simulink model "boostConverter"  (R2021a)
settings: Solver=VariableStepAuto  StartTime=0.0  StopTime=2  RelTol=1e-3
model workspace (MAT data in the model file):
  C = Simulink.Parameter
  C.Value = 0.01
  C.DataType = 'auto'
  C.Dimensions = [1 1]
  L = Simulink.Parameter
  L.Value = 1e-05
  L.DataType = 'auto'
  L.Dimensions = [1 1]
  R = Simulink.Parameter
  R.Value = 10
  R.DataType = 'auto'
  R.Dimensions = [1 1]
libraries: spsSeriesRLCBranchLib x6, spsCurrentMeasurementLib x5, spsMosfetLib x3, spsVoltageMeasurementLib x3, spsControlledVoltageSourceLib x2, spsMeanLib x2, spsDiodeLib x1, simulink x1, spspowerguiLib x1
settings Model: Creator=User  LastModifiedBy=User

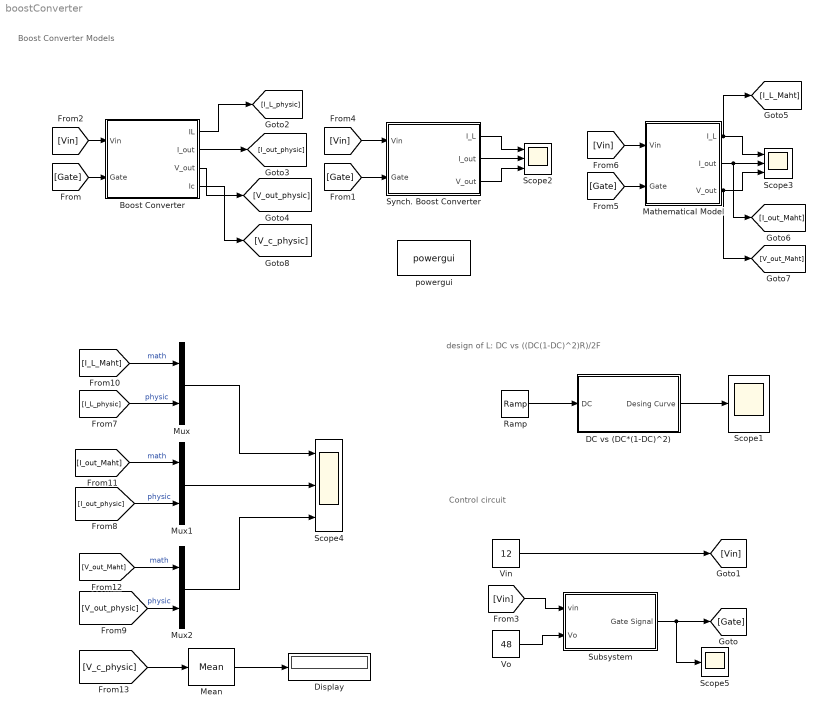
== system boostConverter ==
  note: Control circuit
  note: Boost Converter Models
  note: design of L: DC vs ((DC(1-DC)^2)R)/2F
  " DC vs (DC*(1-DC)^2) " : Subsystem  mask{F=50000, R=R, L=L}
  Boost Converter : Subsystem
  Display : Display
  Mathematical Model : Subsystem
  Mean : spsMeanLib/Mean  Freq=60  Vinit=0  Ts=0
  Mux : Mux  Inputs=2
  Mux1 : Mux  Inputs=2
  Mux2 : Mux  Inputs=2
  Ramp : simulink/Sources/Ramp  slope=1  start=0  InitialOutput=0
  Scope1 : Scope
  Scope2 : Scope  NumInputPorts=3
  Scope3 : Scope  NumInputPorts=3
  Scope4 : Scope  NumInputPorts=3
  Scope5 : Scope
  Subsystem : Subsystem
  Synch. Boost Converter : Subsystem
  Vin : Constant  Value=12
  Vo : Constant  Value=48
  powergui : spspowerguiLib/powergui  Priority=1  SimulationMode=Continuous  SampleTime=50e-6  frequency=60  Iterations=50  frequencyindice=0  Pbase=100e6  ErrMax=1e-4  UnitsV=kV  UnitsW=MW  buscounter=0  FunctionMessages=off  echomessages=off  EnableUseOfTLC=off  CurrentSourceSwitches=off  DisableSnubberDevices=on  DisableRonSwitches=off  DisableVfSwitches=off  DisplayEquations=off  AutomaticDiscreteSolvers=off  SolverType=Tustin/Backward Euler (TBE)  Interpol=off  ExternalGateDelay=off  methode=off  Ts=100  x0status=blocks  SPID=on  SwTol=0  HookPort=off  NonlinearTolerance=1e-4  nMaxIteration=100  ContinueOnMaxIteration=off  RestoreLinks=warning  ResistiveCurrentMeasurement=off  Frange=[0:2:500]  Ylog=off  Xlog=on  ShowGrid=off  save=off  variable=ZData  structure=0  ZoomFFT=off  StartTime=0.0  cycles=1  DisplayStyle=1  fundamental=60  FreqAxis=off  MaxFrequency=1000  frequencyindicesteady=1  RmsSteady=1  display=off
  wires:
  Vo/1 -> Subsystem/2(Vo)
  [Gate] -> Boost Converter/2(Gate)
  Ramp/1 -> " DC vs (DC*(1-DC)^2) "/1(DC)
  " DC vs (DC*(1-DC)^2) "/1(Desing Curve) -> Scope1/1
  Boost Converter/1(IL) -> [I_L_physic]
  [Gate] -> Synch. Boost Converter/2(Gate)
  Synch. Boost Converter/2(I_out) -> Scope2/2
  Synch. Boost Converter/1(I_L) -> Scope2/1
  Synch. Boost Converter/3(V_out) -> Scope2/3
  Vin/1 -> [Vin]
  [Vin] -> Boost Converter/1(Vin)
  [Vin] -> Subsystem/1(vin)
  [Vin] -> Synch. Boost Converter/1(Vin)
  [Gate] -> Mathematical Model/2(Gate)
  [Vin] -> Mathematical Model/1(Vin)
  Boost Converter/2(I_out) -> [I_out_physic]
  Boost Converter/3(V_out) -> [V_out_physic]
  Mathematical Model/1(I_L) -> [I_L_Maht], Scope3/1
  Mathematical Model/2(I_out) -> [I_out_Maht], Scope3/2
  Mathematical Model/3(V_out) -> [V_out_Maht], Scope3/3
  [I_L_Maht] -> Mux/1  "math"
  [I_L_physic] -> Mux/2  "physic"
  [I_out_Maht] -> Mux1/1  "math"
  [I_out_physic] -> Mux1/2  "physic"
  [V_out_Maht] -> Mux2/1  "math"
  [V_out_physic] -> Mux2/2  "physic"
  Mux/1 -> Scope4/1
  Mux1/1 -> Scope4/2
  Mux2/1 -> Scope4/3
  Subsystem/1(Gate Signal) -> Scope5/1, [Gate]
  Boost Converter/4(Ic) -> [V_c_physic]
  [V_c_physic] -> Mean/1
  Mean/1 -> Display/1

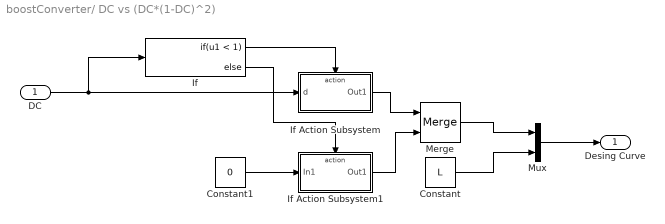
== system boostConverter/ DC vs (DC*(1-DC)^2)  ==
  DC : Inport
  Constant : Constant  Value=L
  Constant1 : Constant  Value=0
  If : If  IfExpression=u1 < 1
  If Action Subsystem : Subsystem  TreatAsAtomicUnit=on
  If Action Subsystem1 : Subsystem  TreatAsAtomicUnit=on
  Merge : Merge
  Mux : Mux  Inputs=2
  Desing Curve : Outport
  wires:
  Constant1/1 -> If Action Subsystem1/1(In1)
  If Action Subsystem/1(Out1) -> Merge/1
  If Action Subsystem1/1(Out1) -> Merge/2
  If/1 -> If Action Subsystem/Action
  DC/1 -> If/1, If Action Subsystem/1(d)
  If/2 -> If Action Subsystem1/Action
  Merge/1 -> Mux/1
  Constant/1 -> Mux/2
  Mux/1 -> Desing Curve/1

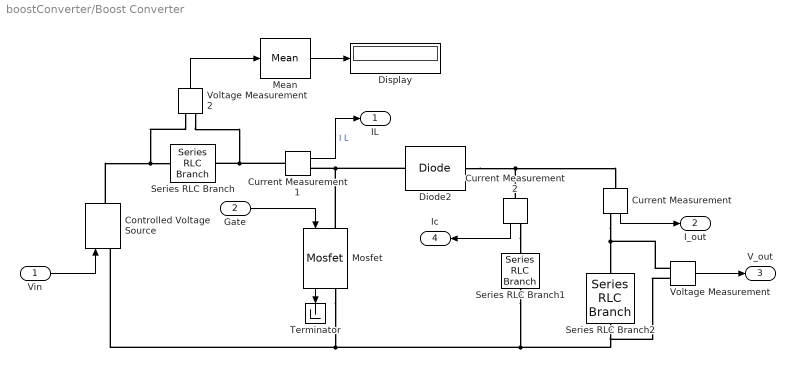
== system boostConverter/Boost Converter ==
  Vin : Inport
  Gate : Inport  Port=2
  Controlled Voltage Source : spsControlledVoltageSourceLib/Controlled Voltage Source  Initialize=on  Source_Type=AC  Amplitude=0  Phase=0  Frequency=0  Measurements=None
  Current Measurement : spsCurrentMeasurementLib/Current Measurement  PhasorSimulation=off  OutputType=Complex  PSBequivalent=0
  Current Measurement1 : spsCurrentMeasurementLib/Current Measurement  PhasorSimulation=off  OutputType=Complex  PSBequivalent=0
  Current Measurement2 : spsCurrentMeasurementLib/Current Measurement  PhasorSimulation=off  OutputType=Complex  PSBequivalent=0
  Diode2 : spsDiodeLib/Diode  Ron=0.001  Lon=0  Vf=0.8  IC=0  UseSnubber=0  Rs=500  Cs=250e-9  Measurements=off
  Display : Display
  Mean : spsMeanLib/Mean  Freq=60  Vinit=0  Ts=0
  Mosfet : spsMosfetLib/Mosfet  Ron=0.1  Lon=0  Rd=0.01  Vfd=0  IC=0  Rs=1e5  Cs=inf  Measurements=on
  Series RLC Branch : spsSeriesRLCBranchLib/Series RLC Branch  LConnTagsString=__new0  RConnTagsString=__new0  BranchType=L  Resistance=1  Inductance=L  SetiL0=off  InitialCurrent=0  Capacitance=1e-6  Setx0=off  InitialVoltage=0  Measurements=None
  Series RLC Branch1 : spsSeriesRLCBranchLib/Series RLC Branch  LConnTagsString=__new0  RConnTagsString=__new0  BranchType=C  Resistance=1  Inductance=1e-3  SetiL0=off  InitialCurrent=0  Capacitance=C  Setx0=off  InitialVoltage=0  Measurements=None
  Series RLC Branch2 : spsSeriesRLCBranchLib/Series RLC Branch  LConnTagsString=__new0  RConnTagsString=__new0  BranchType=R  Resistance=R  Inductance=1e-3  SetiL0=off  InitialCurrent=0  Capacitance=1e-6  Setx0=off  InitialVoltage=0  Measurements=None
  Terminator : Terminator
  Voltage Measurement : spsVoltageMeasurementLib/Voltage Measurement  PhasorSimulation=off  OutputType=Complex  PSBequivalent=0
  Voltage Measurement2 : spsVoltageMeasurementLib/Voltage Measurement  PhasorSimulation=off  OutputType=Complex  PSBequivalent=0
  IL : Outport
  I_out : Outport  Port=2
  V_out : Outport  Port=3
  Ic : Outport  Port=4
  wires:
  Gate/1 -> Mosfet/1
  Current Measurement/1 -> I_out/1
  Mosfet/1 -> Terminator/1
  Current Measurement1/1 -> IL/1  "I L"
  Voltage Measurement/1 -> V_out/1
  Vin/1 -> Controlled Voltage Source/1
  Current Measurement2/1 -> Ic/1
  Voltage Measurement2/1 -> Mean/1
  Mean/1 -> Display/1
  connections:
  Voltage Measurement/LConn2 -- Series RLC Branch2/RConn1 -- Series RLC Branch1/RConn1 -- Controlled Voltage Source/LConn1 -- Mosfet/RConn1
  Mosfet/LConn1 -- Diode2/LConn1 -- Current Measurement1/RConn1
  Diode2/RConn1 -- Current Measurement2/LConn1 -- Current Measurement/LConn1
  Current Measurement/RConn1 -- Series RLC Branch2/LConn1 -- Voltage Measurement/LConn1
  Current Measurement1/LConn1 -- Voltage Measurement2/LConn2 -- Series RLC Branch/RConn1
  Controlled Voltage Source/RConn1 -- Voltage Measurement2/LConn1 -- Series RLC Branch/LConn1
  Current Measurement2/RConn1 -- Series RLC Branch1/LConn1

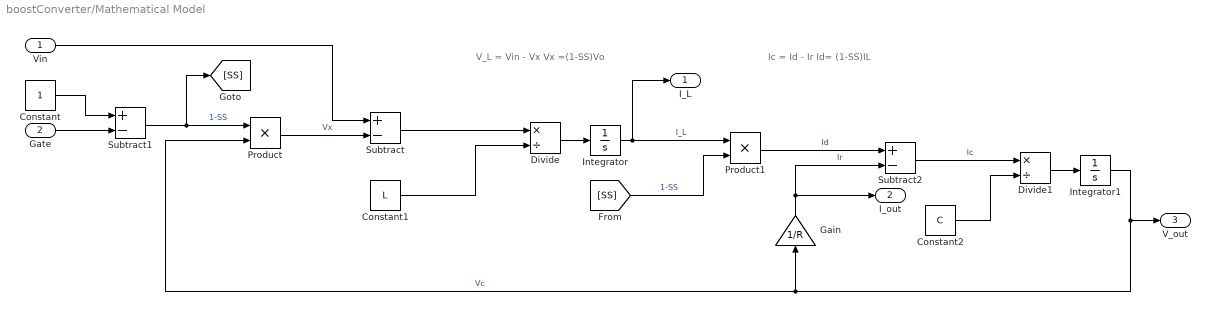
== system boostConverter/Mathematical Model ==
  note: Ic = Id - Ir
      | Id= (1-SS)IL
  note: V_L = Vin - Vx
      | Vx   =(1-SS)Vo
  Vin : Inport
  Gate : Inport  Port=2
  Constant : Constant
  Constant1 : Constant  Value=L
  Constant2 : Constant  Value=C
  Divide : Product  Inputs=*/
  Divide1 : Product  Inputs=*/
  Gain : Gain  Gain=1/R
  Integrator : Integrator  LimitOutput=on  LowerSaturationLimit=0
  Integrator1 : Integrator  LimitOutput=on  LowerSaturationLimit=0
  Product : Product
  Product1 : Product
  Subtract : Sum  Inputs=+-
  Subtract1 : Sum  Inputs=+-
  Subtract2 : Sum  Inputs=+-
  I_L : Outport
  I_out : Outport  Port=2
  V_out : Outport  Port=3
  wires:
  Vin/1 -> Subtract/1
  Product/1 -> Subtract/2  "Vx"
  Gate/1 -> Subtract1/2
  Constant/1 -> Subtract1/1
  Subtract1/1 -> [SS], Product/1  "1-SS"
  Subtract/1 -> Divide/1
  Constant1/1 -> Divide/2
  Divide/1 -> Integrator/1
  [SS] -> Product1/2  "1-SS"
  Product1/1 -> Subtract2/1  "Id"
  Gain/1 -> I_out/1, Subtract2/2  "Ir"
  Subtract2/1 -> Divide1/1  "Ic"
  Constant2/1 -> Divide1/2
  Divide1/1 -> Integrator1/1
  Integrator/1 -> Product1/1, I_L/1  "I_L"
  Integrator1/1 -> V_out/1, Gain/1, Product/2  "Vc"

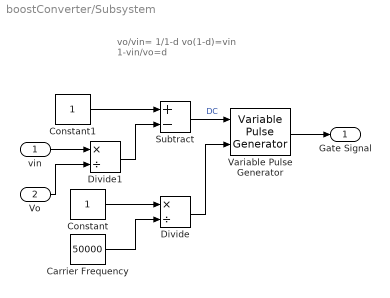
== system boostConverter/Subsystem ==
  note: vo/vin= 1/1-d
      | vo(1-d)=vin
      | 1-vin/vo=d
  vin : Inport
  Vo : Inport  Port=2
  Carrier Frequency : Constant  Value=50000
  Constant : Constant
  Constant1 : Constant
  Divide : Product  Inputs=*/
  Divide1 : Product  Inputs=*/
  Subtract : Sum  Inputs=+-
  Variable Pulse Generator : VariablePulseGenerator  SampleTime=0.1
  Gate Signal : Outport
  wires:
  Divide/1 -> Variable Pulse Generator/2
  Vo/1 -> Divide1/2
  Variable Pulse Generator/1 -> Gate Signal/1
  Carrier Frequency/1 -> Divide/2
  Constant/1 -> Divide/1
  Divide1/1 -> Subtract/2
  vin/1 -> Divide1/1
  Constant1/1 -> Subtract/1
  Subtract/1 -> Variable Pulse Generator/1  "DC"

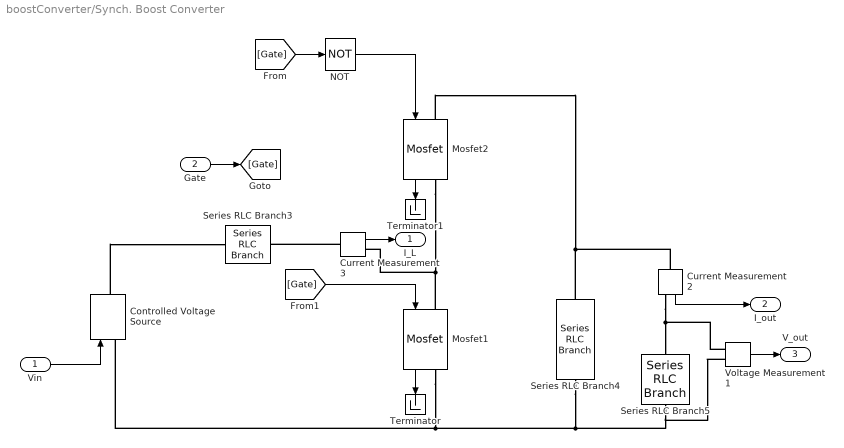
== system boostConverter/Synch. Boost Converter ==
  Vin : Inport
  Gate : Inport  Port=2
  Controlled Voltage Source : spsControlledVoltageSourceLib/Controlled Voltage Source  Initialize=on  Source_Type=AC  Amplitude=0  Phase=0  Frequency=0  Measurements=None
  Current Measurement2 : spsCurrentMeasurementLib/Current Measurement  PhasorSimulation=off  OutputType=Complex  PSBequivalent=0
  Current Measurement3 : spsCurrentMeasurementLib/Current Measurement  PhasorSimulation=off  OutputType=Complex  PSBequivalent=0
  Mosfet1 : spsMosfetLib/Mosfet  Ron=0.1  Lon=0  Rd=0.01  Vfd=0  IC=0  Rs=1e5  Cs=inf  Measurements=on
  Mosfet2 : spsMosfetLib/Mosfet  Ron=0.1  Lon=0  Rd=0.01  Vfd=0  IC=0  Rs=1e5  Cs=inf  Measurements=on
  NOT : Logic  Operator=NOT  IconShape=distinctive  AllPortsSameDT=off  OutDataTypeStr=boolean
  Series RLC Branch3 : spsSeriesRLCBranchLib/Series RLC Branch  LConnTagsString=__new0  RConnTagsString=__new0  BranchType=L  Resistance=1  Inductance=100e-3  SetiL0=off  InitialCurrent=0  Capacitance=1e-6  Setx0=off  InitialVoltage=0  Measurements=None
  Series RLC Branch4 : spsSeriesRLCBranchLib/Series RLC Branch  LConnTagsString=__new0  RConnTagsString=__new0  BranchType=C  Resistance=1  Inductance=1e-3  SetiL0=off  InitialCurrent=0  Capacitance=10e-3  Setx0=off  InitialVoltage=0  Measurements=None
  Series RLC Branch5 : spsSeriesRLCBranchLib/Series RLC Branch  LConnTagsString=__new0  RConnTagsString=__new0  BranchType=R  Resistance=10  Inductance=1e-3  SetiL0=off  InitialCurrent=0  Capacitance=1e-6  Setx0=off  InitialVoltage=0  Measurements=None
  Terminator : Terminator
  Terminator1 : Terminator
  Voltage Measurement1 : spsVoltageMeasurementLib/Voltage Measurement  PhasorSimulation=off  OutputType=Complex  PSBequivalent=0
  I_L : Outport
  I_out : Outport  Port=2
  V_out : Outport  Port=3
  wires:
  Voltage Measurement1/1 -> V_out/1
  NOT/1 -> Mosfet2/1
  Current Measurement2/1 -> I_out/1
  Current Measurement3/1 -> I_L/1
  Mosfet1/1 -> Terminator/1
  Mosfet2/1 -> Terminator1/1
  Gate/1 -> [Gate]
  [Gate] -> NOT/1
  [Gate] -> Mosfet1/1
  Vin/1 -> Controlled Voltage Source/1
  connections:
  Mosfet1/RConn1 -- Controlled Voltage Source/LConn1 -- Series RLC Branch4/RConn1 -- Series RLC Branch5/RConn1 -- Voltage Measurement1/LConn2
  Controlled Voltage Source/RConn1 -- Series RLC Branch3/LConn1
  Mosfet1/LConn1 -- Mosfet2/RConn1 -- Current Measurement3/RConn1
  Series RLC Branch4/LConn1 -- Mosfet2/LConn1 -- Current Measurement2/LConn1
  Current Measurement2/RConn1 -- Voltage Measurement1/LConn1 -- Series RLC Branch5/LConn1
  Current Measurement3/LConn1 -- Series RLC Branch3/RConn1

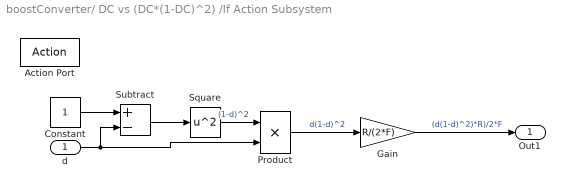
== system boostConverter/ DC vs (DC*(1-DC)^2) /If Action Subsystem ==
  d : Inport
  Action Port : ActionPort  ActionPortLabel=if(u1 < 1)
  Constant : Constant
  Gain : Gain  Gain=R/(2*F)
  Product : Product
  Square : Math  Operator=square  SaturateOnIntegerOverflow=on
  Subtract : Sum  Inputs=+-
  Out1 : Outport
  wires:
  d/1 -> Product/2, Subtract/2
  Subtract/1 -> Square/1
  Product/1 -> Gain/1  "d(1-d)^2"
  Square/1 -> Product/1  "(1-d)^2"
  Constant/1 -> Subtract/1
  Gain/1 -> Out1/1  "(d(1-d)^2)*R)/2*F"

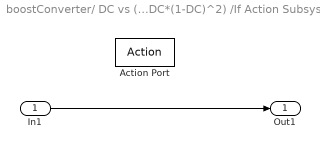
== system boostConverter/ DC vs (DC*(1-DC)^2) /If Action Subsystem1 ==
  In1 : Inport
  Action Port : ActionPort  ActionPortLabel=else
  Out1 : Outport
  wires:
  In1/1 -> Out1/1
